simulink model "PID_controller_implementation"  (R2023b)
settings: Solver=ode8  StartTime=0.0  StopTime=20  FixedStep=0.005  RelTol=1e-3
settings Model: Creator=suvo  LastModifiedBy=suvo
settings SolverCC: AlgebraicLoopSolver=TrustRegion
settings DataIOCC: ReturnWorkspaceOutputs=off
settings DebuggingCC: UnconnectedInputMsg=warning  UnconnectedOutputMsg=warning  UnconnectedLineMsg=warning
settings ModelReferenceCC: EnableRefExpFcnMdlSchedulingChecks=on

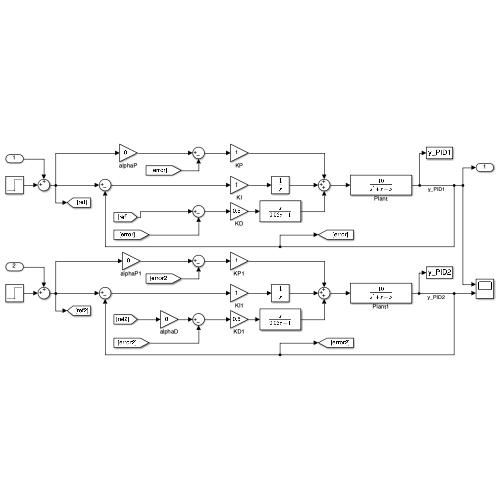
[thumbnail: Simulink's stored preview of the top-level diagram]
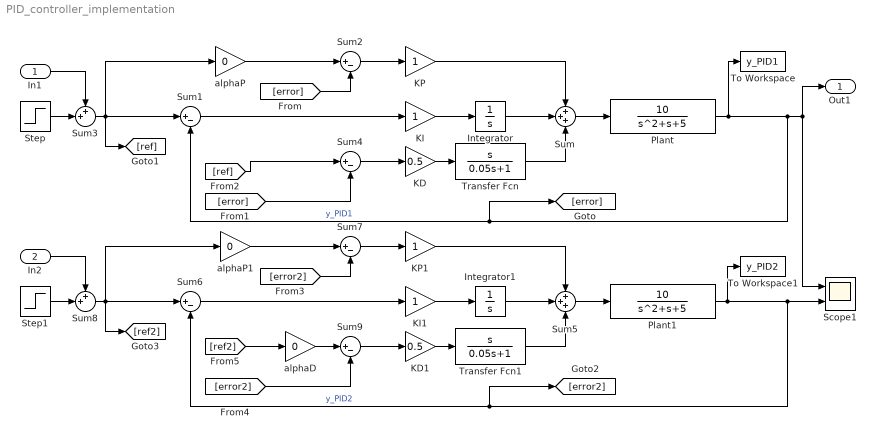
== system PID_controller_implementation ==
  In1 : Inport
  In2 : Inport  Port=2
  Integrator : Integrator
  Integrator1 : Integrator
  KD : Gain  Gain=0.5
  KD1 : Gain  Gain=0.5
  KI : Gain
  KI1 : Gain
  KP : Gain
  KP1 : Gain
  Plant : TransferFcn  Numerator=10  Denominator=[1 1 5]
  Plant1 : TransferFcn  Numerator=10  Denominator=[1 1 5]
  Scope1 : Scope  NumInputPorts=2
  Step : Step  SampleTime=0
  Step1 : Step  SampleTime=0
  Sum : Sum  Inputs=+++
  Sum{1..2,4,6..7,9} (6 alike) : Sum  Inputs=|+-
  Sum3 : Sum  Inputs=++|
  Sum5 : Sum  Inputs=+++
  Sum8 : Sum  Inputs=++|
  To Workspace : ToWorkspace  VariableName=y_PID1  SaveFormat=Timeseries  SampleTime=-1
  To Workspace1 : ToWorkspace  VariableName=y_PID2  SaveFormat=Timeseries  SampleTime=-1
  Transfer Fcn : TransferFcn  Numerator=[1 0]  Denominator=[0.05 1]
  Transfer Fcn1 : TransferFcn  Numerator=[1 0]  Denominator=[0.05 1]
  alphaD : Gain  Gain=0
  alphaP : Gain  Gain=0
  alphaP1 : Gain  Gain=0
  Out1 : Outport
  wires:
  KI/1 -> Integrator/1
  Sum1/1 -> KI/1
  Plant/1 -> To Workspace/1, Scope1/1, Out1/1, Sum1/2, [error]  "y_PID1"
  Sum3/1 -> alphaP/1, Sum1/1, [ref]
  Sum2/1 -> KP/1
  KP/1 -> Sum/1
  Integrator/1 -> Sum/2
  Sum/1 -> Plant/1
  In1/1 -> Sum3/1
  Step/1 -> Sum3/2
  [error] -> Sum2/2
  KD/1 -> Transfer Fcn/1
  Transfer Fcn/1 -> Sum/3
  Sum4/1 -> KD/1
  [error] -> Sum4/2
  [ref] -> Sum4/1
  Transfer Fcn1/1 -> Sum5/3
  [error2] -> Sum7/2
  KP1/1 -> Sum5/1
  Integrator1/1 -> Sum5/2
  Sum9/1 -> KD1/1
  Sum8/1 -> alphaP1/1, Sum6/1, [ref2]
  Sum7/1 -> KP1/1
  In2/1 -> Sum8/1
  Step1/1 -> Sum8/2
  KI1/1 -> Integrator1/1
  Sum5/1 -> Plant1/1
  Sum6/1 -> KI1/1
  KD1/1 -> Transfer Fcn1/1
  Plant1/1 -> To Workspace1/1, Sum6/2, [error2], Scope1/2  "y_PID2"
  [error2] -> Sum9/2
  [ref2] -> alphaD/1
  alphaP1/1 -> Sum7/1
  alphaP/1 -> Sum2/1
  alphaD/1 -> Sum9/1
